simulink model "probe_6"  (R2020b)
settings: Solver=VariableStepAuto  StartTime=0.0  StopTime=10.0  RelTol=1e-3
settings Model: Creator=admin  LastModifiedBy=admin

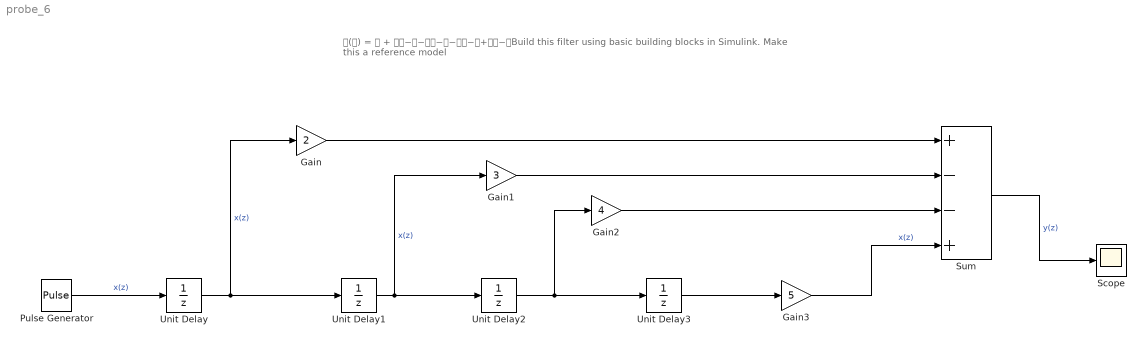
== system probe_6 ==
  note: 𝐇(𝐳) = 𝟏 + 𝟐𝐳−𝟏−𝟑𝐳−𝟐−𝟒𝐳−𝟑+𝟓𝐳−𝟒Build this filter using basic building blocks in Simulink. Make this a reference model
  Gain : Gain  Gain=2
  Gain1 : Gain  Gain=3
  Gain2 : Gain  Gain=4
  Gain3 : Gain  Gain=5
  Pulse Generator : DiscretePulseGenerator  PulseType=Time based  Period=10  PulseWidth=5
  Scope : Scope
  Sum : Sum  Inputs=+--+
  Unit Delay{,1..3} (4 alike) : UnitDelay  SampleTime=-1  HasFrameUpgradeWarning=on
  wires:
  Pulse Generator/1 -> Unit Delay/1  "x(z)"
  Unit Delay/1 -> Gain/1, Unit Delay1/1  "x(z)"
  Unit Delay1/1 -> Unit Delay2/1, Gain1/1  "x(z)"
  Unit Delay2/1 -> Gain2/1, Unit Delay3/1
  Unit Delay3/1 -> Gain3/1
  Sum/1 -> Scope/1  "y(z)"
  Gain/1 -> Sum/1
  Gain1/1 -> Sum/2
  Gain2/1 -> Sum/3
  Gain3/1 -> Sum/4  "x(z)"
